simulink model "mechatronik_projekt_simulink_regler_work02"  (Simulink 7.6)
settings: Solver=ode45  StartTime=0.0  StopTime=10  MaxStep=1e-2  RelTol=1e-3
libraries: simulink x3
settings Model: Creator=MATLAB-Benutzer  LastModifiedBy=MATLAB-Benutzer
settings OptimizationCC: InitFltsAndDblsToZero=on
settings DebuggingCC: SaveWithParameterizedLinksMsg=none  SignalResolutionControl=TryResolveAllWithWarning  MultiTaskDSMMsg=warning  MultiTaskCondExecSysMsg=none  StrictBusMsg=Warning
settings SFSimCC: SimParseCustomCode=off
settings RTWCC: IncludeERTFirstTime=on
settings GRTTargetCC: TargetFcnLib=ansi_tfl_tmw.mat

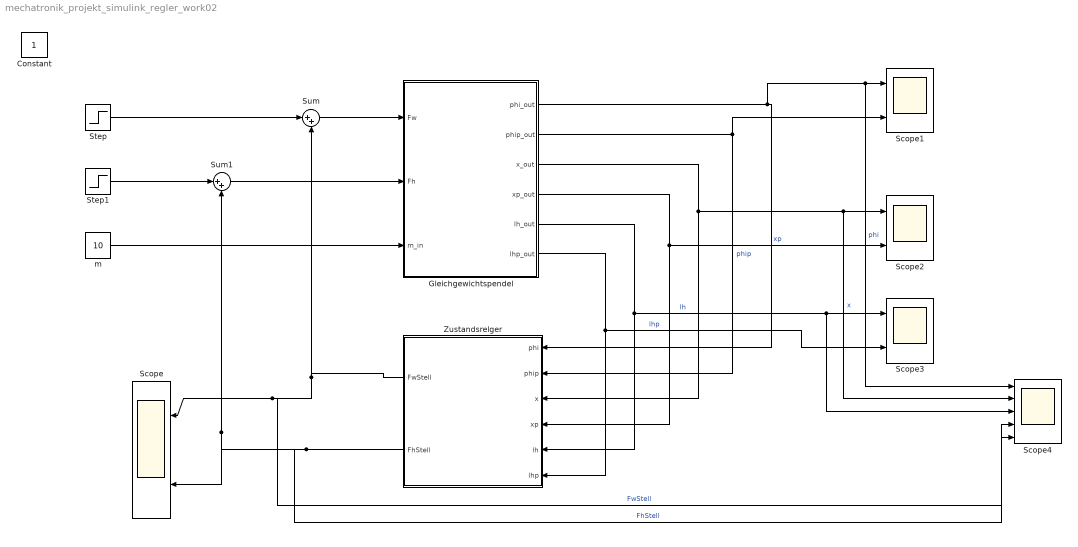
== system mechatronik_projekt_simulink_regler_work02 ==
  Gleichgewichtspendel : Subsystem
  Scope{,1..3} (4 alike) : Scope  NumInputPorts=2
      Scope settings: TickLabels=on  YMin=-5~-5  YMax=5~5
      Scope1 settings: TickLabels=on  YMin=-5~-5  YMax=5~5
      Scope2 settings: TickLabels=on  YMin=-0.025~-0.2  YMax=0.525~0.5  SaveName=ScopeData2
      Scope3 settings: TickLabels=on  YMin=-5~-5  YMax=5~5  SaveName=ScopeData3
  Scope4 : Scope  NumInputPorts=5
      settings: TickLabels=on  TimeRange=4  YMin=-2~-10~0~-5000~-20  YMax=2~10~4~4000~20  SaveName=ScopeData4  MaxDataPoints=50000
  Step : Step  Time=0.1  Before=-1  After=0  SampleTime=0
  Step1 : Step  Time=0  After=0  SampleTime=0
  Sum : Sum  Inputs=|++
  Sum1 : Sum  Inputs=|++
  Zustandsrelger : Stateflow chart  TreatAsAtomicUnit=on
  m : Constant  Value=10
  Constant : Constant  IOType=siggen
  wires:
  Gleichgewichtspendel/1(phi_out) -> Zustandsrelger/1(phi), Scope1/1, Scope4/1  "phi"
  Gleichgewichtspendel/2(phip_out) -> Zustandsrelger/2(phip), Scope1/2  "phip"
  Gleichgewichtspendel/3(x_out) -> Zustandsrelger/3(x), Scope2/1, Scope4/2  "x"
  Gleichgewichtspendel/4(xp_out) -> Zustandsrelger/4(xp), Scope2/2  "xp"
  Gleichgewichtspendel/5(lh_out) -> Zustandsrelger/5(lh), Scope3/1, Scope4/3  "lh"
  Gleichgewichtspendel/6(lhp_out) -> Zustandsrelger/6(lhp), Scope3/2  "lhp"
  m/1 -> Gleichgewichtspendel/3(m_in)
  Zustandsrelger/1(FwStell) -> Sum/2, Scope/1, Scope4/4  "FwStell"
  Zustandsrelger/2(FhStell) -> Sum1/2, Scope/2, Scope4/5  "FhStell"
  Step1/1 -> Sum1/1
  Sum1/1 -> Gleichgewichtspendel/2(Fh)
  Sum/1 -> Gleichgewichtspendel/1(Fw)
  Step/1 -> Sum/1

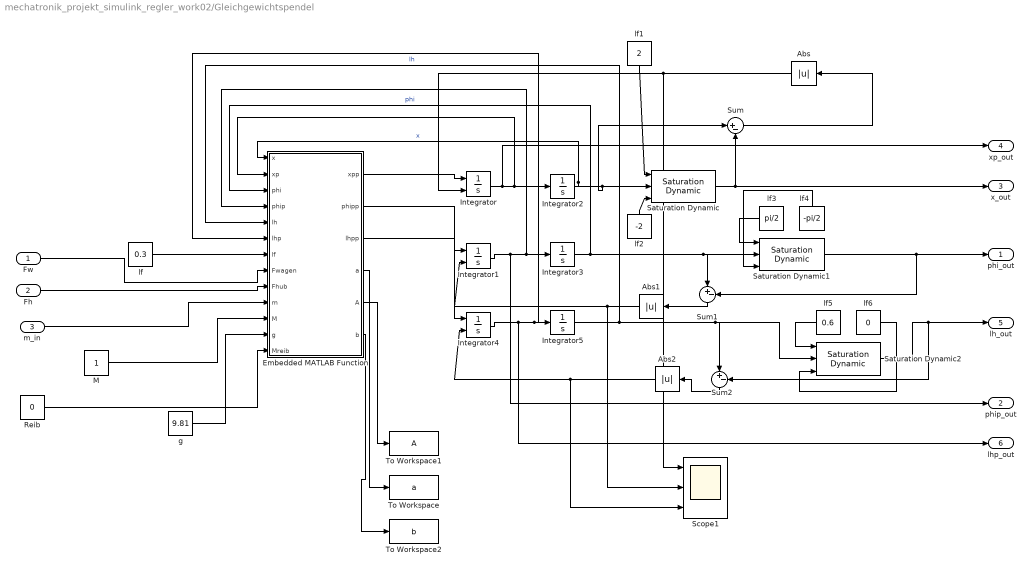
== system mechatronik_projekt_simulink_regler_work02/Gleichgewichtspendel ==
  Fw : Inport
  Fh : Inport  Port=2
  m_in : Inport  Port=3
  Abs : Abs
  Abs1 : Abs
  Abs2 : Abs
  Embedded MATLAB Function : Stateflow chart  TreatAsAtomicUnit=on
  Integrator : Integrator  ExternalReset=rising
  Integrator1 : Integrator  ExternalReset=level
  Integrator2 : Integrator  UpperSaturationLimit=1  LowerSaturationLimit=-1
  Integrator3 : Integrator  UpperSaturationLimit=pi/2  LowerSaturationLimit=-pi/2
  Integrator4 : Integrator  ExternalReset=rising
  Integrator5 : Integrator  InitialCondition=0.3  UpperSaturationLimit=2  LowerSaturationLimit=0
  M : Constant
  Reib : Constant  Value=0
  Saturation Dynamic : simulink/Discontinuities/Saturation Dynamic  SystemSampleTime=-1  OutMin=[]  OutMax=[]  OutDataTypeStr=Inherit: Same as second input  OutDataType=fixdt(1, 16)  OutScaling=2^-10  DoSatur=off
  Saturation Dynamic1 : simulink/Discontinuities/Saturation Dynamic  SystemSampleTime=-1  OutMin=[]  OutMax=[]  OutDataTypeStr=Inherit: Same as second input  OutDataType=fixdt(1, 16)  OutScaling=2^-10  DoSatur=off
  Saturation Dynamic2 : simulink/Discontinuities/Saturation Dynamic  SystemSampleTime=-1  OutMin=[]  OutMax=[]  OutDataTypeStr=Inherit: Same as second input  OutDataType=fixdt(1, 16)  OutScaling=2^-10  DoSatur=off
  Scope1 : Scope  NumInputPorts=3
      settings: TickLabels=on  YMin=-5~-5~-5  YMax=5~5~5  SaveName=ScopeData5
  Sum : Sum  Inputs=|+-
  Sum1 : Sum  Inputs=|+-
  Sum2 : Sum  Inputs=|+-
  To Workspace : ToWorkspace  VariableName=a  SampleTime=-1  SaveFormat=Structure
  To Workspace1 : ToWorkspace  VariableName=A  SampleTime=-1  SaveFormat=Structure
  To Workspace2 : ToWorkspace  VariableName=b  SampleTime=-1  SaveFormat=Structure
  g : Constant  Value=9.81
  lf : Constant  Value=0.3
  lf1 : Constant  Value=2
  lf2 : Constant  Value=-2
  lf3 : Constant  Value=pi/2
  lf4 : Constant  Value=-pi/2
  lf5 : Constant  Value=0.6
  lf6 : Constant  Value=0
  phi_out : Outport
  phip_out : Outport  Port=2
  x_out : Outport  Port=3
  xp_out : Outport  Port=4
  lh_out : Outport  Port=5
  lhp_out : Outport  Port=6
  wires:
  Fw/1 -> Embedded MATLAB Function/8(Fwagen)
  Fh/1 -> Embedded MATLAB Function/9(Fhub)
  M/1 -> Embedded MATLAB Function/11(M)
  m_in/1 -> Embedded MATLAB Function/10(m)
  g/1 -> Embedded MATLAB Function/12(g)
  lf/1 -> Embedded MATLAB Function/7(lf)
  Integrator5/1 -> Embedded MATLAB Function/5(lh), Saturation Dynamic2/2, Sum2/1  "lh"
  Integrator3/1 -> Embedded MATLAB Function/3(phi), Saturation Dynamic1/2, Sum1/1  "phi"
  Integrator2/1 -> Saturation Dynamic/2, Sum/1, Embedded MATLAB Function/1(x)  "x"
  Embedded MATLAB Function/3(lhpp) -> Integrator4/1
  Embedded MATLAB Function/2(phipp) -> Integrator1/1
  Embedded MATLAB Function/1(xpp) -> Integrator/1
  Integrator4/1 -> Integrator5/1, Embedded MATLAB Function/6(lhp), lhp_out/1
  Integrator1/1 -> Integrator3/1, Embedded MATLAB Function/4(phip), phip_out/1
  Integrator/1 -> Integrator2/1, Embedded MATLAB Function/2(xp), xp_out/1
  Reib/1 -> Embedded MATLAB Function/13(Mreib)
  Saturation Dynamic/1 -> x_out/1, Sum/2
  lf1/1 -> Saturation Dynamic/1
  Sum/1 -> Abs/1
  Abs/1 -> Integrator/2, Scope1/1
  lf2/1 -> Saturation Dynamic/3
  Saturation Dynamic1/1 -> phi_out/1, Sum1/2
  lf3/1 -> Saturation Dynamic1/1
  lf4/1 -> Saturation Dynamic1/3
  Sum1/1 -> Abs1/1
  Abs1/1 -> Integrator1/2, Scope1/2
  Saturation Dynamic2/1 -> lh_out/1, Sum2/2
  lf5/1 -> Saturation Dynamic2/1
  lf6/1 -> Saturation Dynamic2/3
  Sum2/1 -> Abs2/1
  Abs2/1 -> Integrator4/2, Scope1/3
  Embedded MATLAB Function/4(a) -> To Workspace/1
  Embedded MATLAB Function/5(A) -> To Workspace1/1
  Embedded MATLAB Function/6(b) -> To Workspace2/1

== matlab function Zustandsrelger ==
  data: phi input double; FwStell output double; phip input double; x input double; xp input double; lh input double; lhp input double; FhStell output double
function [FwStell, FhStell] = fcn(phi, phip, x, xp, lh, lhp)
% 2D Zustandsregler

% k11 = 25;
% k12 = 60;
% k13 = -4;
k11 = 100;
k12 = 100;
k13 = 0;

k14 = 0;
k15 = 0;
k16 = 0;

k21 = 40;
k22 = 100;
k23 = 0;
k24 = 0;
k25 = 0;
k26 = 10;

lh_soll = 0.3;

FwStell = k11*phi + k12*phip + k13*x + k14*xp + k15*lh + k16*lhp;
FhStell = k21*phi + k22*phip + k23*x + k24*xp + k25*(lh_soll-lh) + k26*lhp;

FwStell = -1 * FwStell;
FhStell = -1 * FhStell;

== matlab function Gleichgewichtspendel/Embedded MATLAB Function ==
  settings: fimath=|
      | fimath(...
      | 'RoundMode', 'floor',...
      | 'OverflowMode', 'wrap',...
      | 'ProductMode', 'KeepLSB', 'ProductWordLength', 32,...
      | 'SumMode', 'KeepLSB', 'SumWordLength', 32,...
      | 'CastBeforeSum', false)
  data: x input double; xp input double; phi input double; xpp output double; phip input double; lh input double; lhp input double; lf input double; Fwagen input double; Fhub input double; m input double; M input double; g input double; phipp output double; lhpp output double; Mreib input double; a output double; A output double; b output double
function [xpp, phipp, lhpp, a, A, b] = pendel (x, xp, phi, phip, lh, lhp, lf,  Fwagen, Fhub, m, M, g, Mreib)
% This block supports an embeddable subset of the MATLAB language.
% See the help menu for details. 

A = [ 13/12 * m * (lf +lh)^2 + m * x ^2, m * (lf + lh), 0  ;...
      m * (lf + lh), m ,0 ;...
      0, 0, m
      ];
  
b1 = Mreib + 1/2 * M * g * (lf + lh) * sin(phi) ...
    - g * m * (-1 * (lf + lh) * sin(phi)  - cos(phi) * x) ...
    - 1/6 * m * (lf + lh) * lhp * phip  ...
    - 2 * m * x *phip * xp  ...   
    - m * lhp * ((lf + lh) * phip + xp) ...
    - m * (lf+lh) *lhp * phip;
   
b2 =  Fwagen + g * m * sin(phi) +m * x * phip^2 - m * lhp * phip ;

b3 =  Fhub  - 1/2 * g * M * cos(phi) - g * m * (cos(phi))...
      + 1/12 * m * (lf+lh) * phip^2 ...
      + m * phip * ((lf + lh) * phip + xp);
  
  
  a = inv(A)* [b1; b2; b3];
  %a = A \ [b1; b2; b3];
  b = [b1; b2; b3];
  
 phipp = a(1);
 xpp   = a(2);
 lhpp  = a(3);
 
 
 
 
 
% Mit Cos in ursprungs Formel.
% ============================ 
%b1 = Mreib + 1/2 * M * g * (lf + lh) * sin(phi) - g * m * ((lf +lh) * sin(phi) - x * cos(phi)) ...
%    - 1/6 * m * (lf + lh) * lhp * phip - 2 * m * x * phip * xp - m * lhp ...
%     * (lhp + ( lf +lh)*phip + xp) - m * (lf + lh) * lhp * phip;
%b2 =  Fwagen + g * m * sin(phi) + m * x * phip^2 - m *( lhp * phip);
%b3 =  Fhub - g * m * (1 - cos(phi)) - 1/2 * g* M * (cos(phi)-1)+1/12*m*(lf+lh)*phip^2 ...
%      + m * phip * ( lhp + (lf + lh) * phip +xp) - m * (lhp * phip);
 
% ---------------------------------------------------------------------
 
 
 
%b1 =  Mreib + 1/2 * M * (lf + lh) * sin(phi) - g * m * ((lf +lh) * sin(phi) - x * cos(phi)) ...
%      - 1/6 * m * (lf + lh) * lhp * phip - 2 * m * x * phip * xp - m *lhp ...
%      * (lhp + ( lf +lh)*phip + xp) - m * (lf + lh) * lhp * phip;

% Original GLeichung  mit 1-cos(phi)
%b3 =  Fhub - g * m * (1-cos(phi)) - 1/2 * M * (cos(phi)-1)+1/12*m*(lf+lh)*phip^2 ...
 % 
 %b3 = g * m *(1-Cos(phi))+1/2 * g M (-1+Cos(phi))-1/12 m (lf+lh) (phip)^2-m (phip) ((lhp)+(lf+lh) (phip)+(xp))+m (lhpp)+m ((lhp) (phip)+(lhpp)+(lf+lh) (phipp)+(xpp))
%    + m * phip * ( lhp + (lf + lh) * phip +xp) -m * (lhp*phip);
